simulink model "PlantModelSim"  (R2020a)
settings: Solver=VariableStepAuto  StartTime=0.0  StopTime=30  RelTol=1e-3
values from neighbouring files (symbols this model uses):
  A = [0  0  0  1  0  0  0  0  0  0  0  0 ... (first row only)    [LQR.m]    (also in LQR_Goal_1.m; Naman_LQR_Working.m; PlantModel.m = [0  0  0  1  0  0  0  0  0  0  0  0;      0  0  0  0  1  0  )
  B = [0      0       0       0 ... (first row only)    [LQR.m]    (also in LQR_Goal_1.m; Naman_LQR_Working.m; PlantModel.m = [0 0 0 0;      0 0 0 0;      0 0 0 0;      0 0 0 0;      0 0)
  C = [1 0 0 0 0 0 0 0 0 0 0 0 ... (first row only)    [LQR.m]    (also in LQR_Goal_1.m; Naman_LQR_Working.m; PlantModel.m = [1 0 0 0 0 0 0 0 0 0 0 0;      0 1 0 0 0 0 0 0 0 0 0 0;     )
  D = zeros(6,4)    [LQR.m]    (also in LQR_Goal_1.m; Naman_LQR_Working.m; PlantModel.m)
  g = 9.81    [LQR.m]    (also in LQR_Goal_1.m; Naman_LQR_Working.m; PlantModel.m)
  initialCondition = [x0, y0, z0, xdot0, ydot0, zdot0, phi0, theta0, psi0, phidot0, thetadot0, psidot0]    [PlantModel.m]
  Ix = 4.856*10^-3    (= 0.004856)    [LQR.m]    (also in LQR_Goal_1.m; Naman_LQR_Working.m; PlantModel.m)
  Iy = 4.856*10^-3    (= 0.004856)    [LQR.m]    (also in LQR_Goal_1.m; Naman_LQR_Working.m; PlantModel.m)
  Iz = 8.801*10^-3    (= 0.008801)    [LQR.m]    (also in LQR_Goal_1.m; Naman_LQR_Working.m; PlantModel.m)
  kdp = 0.1    [PlantModel.m]
  kdps = 0.0486    [PlantModel.m]
  kdt = 0.1    [PlantModel.m]
  kdz = 2.9031    [PlantModel.m]
  kpp = 0.4754    [PlantModel.m]
  kpps = 0.0901    [PlantModel.m]
  kpt = 0.4754    [PlantModel.m]
  kpz = 4.0670    (= 4.067)    [PlantModel.m]
  m = 0.468    [LQR.m]    (also in LQR_Goal_1.m; Naman_LQR_Working.m; PlantModel.m)
  phi0 = X0(7)    [LQR_Goal_1.m]    (also in PlantModel.m = 0)
  phidot0 = X0(10)    [LQR_Goal_1.m]    (also in PlantModel.m = 0)
  psi0 = X0(9)    [LQR_Goal_1.m]    (also in PlantModel.m = 0)
  psidot0 = X0(12)    [LQR_Goal_1.m]    (also in PlantModel.m = 0)
  sysd = c2d(sys, 1/100)    [PlantModel.m]
  theta0 = X0(8)    [LQR_Goal_1.m]    (also in PlantModel.m = 0)
  thetadot0 = X0(11)    [LQR_Goal_1.m]    (also in PlantModel.m = 0)
  x0 = X0(1)    [LQR_Goal_1.m]    (also in PlantModel.m = 0)
  x_d = 0    [LQR.m]    (also in PlantModel.m = 1)
  xdot0 = X0(4)    [LQR_Goal_1.m]    (also in PlantModel.m = 0)
  y0 = X0(2)    [LQR_Goal_1.m]    (also in PlantModel.m = 0)
  y_d = 0    [LQR.m]    (also in PlantModel.m = 1)
  ydot0 = X0(5)    [LQR_Goal_1.m]    (also in PlantModel.m = 0)
  z0 = X0(3)    [LQR_Goal_1.m]    (also in PlantModel.m = 0)
  z_d = 0    [LQR.m]    (also in PlantModel.m = 1)
  zdot0 = X0(6)    [LQR_Goal_1.m]    (also in PlantModel.m = 0)
libraries: simulink x11
settings Model: Creator=Lakshu  LastModifiedBy=Sravan

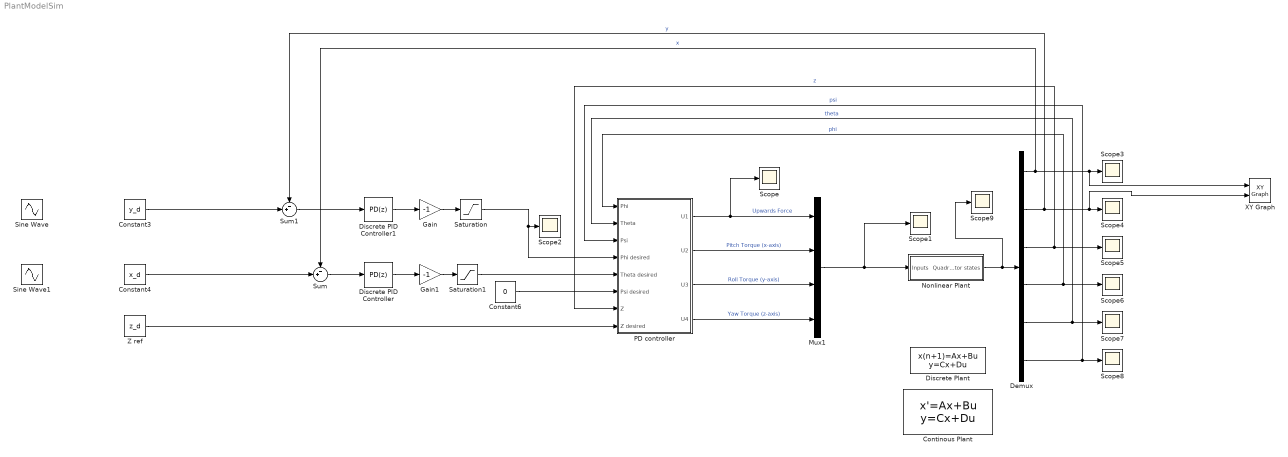
== system PlantModelSim ==
  Constant3 : Constant  Value=y_d
  Constant4 : Constant  Value=x_d
  Constant6 : Constant  Value=0
  Continous Plant : StateSpace  A=A  B=B  C=C  D=D  InitialCondition=initialCondition
  Demux : Demux  Outputs=6
  Discrete PID Controller : simulink/Continuous/PID Controller  Controller=PD  Form=Parallel  TimeDomain=Discrete-time  UseExternalTs=off  SampleTime=-1  IntegratorMethod=Forward Euler  FilterMethod=Forward Euler  ControllerParametersSource=internal  P=-0.0231859221153857  I=-0.00134790003505014  D=-0.0997082443730221  UseFilter=off  N=100  TunerSelectOption=Transfer Function Based (PID Tuner App)  InitialConditionSource=internal  InitialConditionForIntegrator=0  InitialConditionForFilter=0  DifferentiatorICPrevScaledInput=0  ExternalReset=none  TrackingMode=off  Kt=1  LimitOutput=off  UpperSaturationLimit=inf  LowerSaturationLimit=-inf  LinearizeAsGain=off  AntiWindupMode=none  Kb=1  POutMin=[]  POutMax=[]  IOutMin=[]  IOutMax=[]  DOutMin=[]  DOutMax=[]  NOutMin=[]  NOutMax=[]  SumOutMin=[]  SumOutMax=[]  SaturationOutMin=[]  SaturationOutMax=[]  PParamMin=[]  PParamMax=[]  IParamMin=[]  IParamMax=[]  DParamMin=[]  DParamMax=[]  NParamMin=[]  NParamMax=[]  KbParamMin=[]  KbParamMax=[]  KtParamMin=[]  KtParamMax=[]  KbOutMin=[]  KbOutMax=[]  KtOutMin=[]  KtOutMax=[]  IntegratorOutMin=[]  IntegratorOutMax=[]  FilterOutMin=[]  FilterOutMax=[]  SumI1OutMin=[]  SumI1OutMax=[]  SumI2OutMin=[]  SumI2OutMax=[]  SumI3OutMin=[]  SumI3OutMax=[]  SumI4OutMin=[]  SumI4OutMax=[]  SumDOutMin=[]  SumDOutMax=[]  DifferentiatorOutMin=[]  DifferentiatorOutMax=[]  FilterDiffOutCoefMin=[]  FilterDiffOutCoefMax=[]  ReciprocalOutMin=[]  ReciprocalOutMax=[]  SumDenOutMin=[]  SumDenOutMax=[]  SumNumOutMin=[]  SumNumOutMax=[]  DivideOutMin=[]  DivideOutMax=[]  UdiffTsProdOutMin=[]  UdiffTsProdOutMax=[]  NTsProdOutMin=[]  NTsProdOutMax=[]  UintegralTsProdOutMin=[]  UintegralTsProdOutMax=[]  UngainTsProdOutMin=[]  UngainTsProdOutMax=[]  IntegratorContinuousStateAttributes=''  IntegratorStateMustResolveToSignalObject=off  IntegratorRTWStateStorageClass=Auto  FilterContinuousStateAttributes=''  FilterStateMustResolveToSignalObject=off  FilterRTWStateStorageClass=Auto  ParallelPVariant=InternalParameters  IdealPVariant=Disabled  IVariant=Disabled  DVariant=InternalParameters  IntegratorVariant=Disabled  SatVariant=Disabled  AWVariant=Disabled  PCopyVariant=Disabled  TRVariant=Disabled  FdbkBlocksVariant=Forward  IdealPFdbkVariant=Disabled  SatFdbkVariant=Disabled  DerivativeFilterVariant=Differentiator  NVariant=Passthrough  NCopyVariant=Disabled_SignalSpec  FilterICVariant=InternalICsDifferentiator  IntegratorICVariant=Disabled  ExternalResetVariant=Disabled  TRSumVariant=Passthrough  SumFdbkVariant=Disabled  SumVariant=Sum_PD  TsampFilterVariant=InternalTs  TsampNgainVariant=Passthrough  TsampIntegralVariant=Disabled_SignalSpec
  Discrete PID Controller1 : simulink/Continuous/PID Controller  Controller=PD  Form=Parallel  TimeDomain=Discrete-time  UseExternalTs=off  SampleTime=-1  IntegratorMethod=Forward Euler  FilterMethod=Forward Euler  ControllerParametersSource=internal  P=0.0231859221153852  I=0.00134790003505011  D=0.0997082443730201  UseFilter=off  N=100  TunerSelectOption=Transfer Function Based (PID Tuner App)  InitialConditionSource=internal  InitialConditionForIntegrator=0  InitialConditionForFilter=0  DifferentiatorICPrevScaledInput=0  ExternalReset=none  TrackingMode=off  Kt=1  LimitOutput=off  UpperSaturationLimit=inf  LowerSaturationLimit=-inf  LinearizeAsGain=off  AntiWindupMode=none  Kb=1  POutMin=[]  POutMax=[]  IOutMin=[]  IOutMax=[]  DOutMin=[]  DOutMax=[]  NOutMin=[]  NOutMax=[]  SumOutMin=[]  SumOutMax=[]  SaturationOutMin=[]  SaturationOutMax=[]  PParamMin=[]  PParamMax=[]  IParamMin=[]  IParamMax=[]  DParamMin=[]  DParamMax=[]  NParamMin=[]  NParamMax=[]  KbParamMin=[]  KbParamMax=[]  KtParamMin=[]  KtParamMax=[]  KbOutMin=[]  KbOutMax=[]  KtOutMin=[]  KtOutMax=[]  IntegratorOutMin=[]  IntegratorOutMax=[]  FilterOutMin=[]  FilterOutMax=[]  SumI1OutMin=[]  SumI1OutMax=[]  SumI2OutMin=[]  SumI2OutMax=[]  SumI3OutMin=[]  SumI3OutMax=[]  SumI4OutMin=[]  SumI4OutMax=[]  SumDOutMin=[]  SumDOutMax=[]  DifferentiatorOutMin=[]  DifferentiatorOutMax=[]  FilterDiffOutCoefMin=[]  FilterDiffOutCoefMax=[]  ReciprocalOutMin=[]  ReciprocalOutMax=[]  SumDenOutMin=[]  SumDenOutMax=[]  SumNumOutMin=[]  SumNumOutMax=[]  DivideOutMin=[]  DivideOutMax=[]  UdiffTsProdOutMin=[]  UdiffTsProdOutMax=[]  NTsProdOutMin=[]  NTsProdOutMax=[]  UintegralTsProdOutMin=[]  UintegralTsProdOutMax=[]  UngainTsProdOutMin=[]  UngainTsProdOutMax=[]  IntegratorContinuousStateAttributes=''  IntegratorStateMustResolveToSignalObject=off  IntegratorRTWStateStorageClass=Auto  FilterContinuousStateAttributes=''  FilterStateMustResolveToSignalObject=off  FilterRTWStateStorageClass=Auto  ParallelPVariant=InternalParameters  IdealPVariant=Disabled  IVariant=Disabled  DVariant=InternalParameters  IntegratorVariant=Disabled  SatVariant=Disabled  AWVariant=Disabled  PCopyVariant=Disabled  TRVariant=Disabled  FdbkBlocksVariant=Forward  IdealPFdbkVariant=Disabled  SatFdbkVariant=Disabled  DerivativeFilterVariant=Differentiator  NVariant=Passthrough  NCopyVariant=Disabled_SignalSpec  FilterICVariant=InternalICsDifferentiator  IntegratorICVariant=Disabled  ExternalResetVariant=Disabled  TRSumVariant=Passthrough  SumFdbkVariant=Disabled  SumVariant=Sum_PD  TsampFilterVariant=InternalTs  TsampNgainVariant=Passthrough  TsampIntegralVariant=Disabled_SignalSpec
  Discrete Plant : DiscreteStateSpace  A=sysd.A  B=sysd.B  C=sysd.C  D=sysd.D  InitialCondition=initialCondition  SampleTime=.01
  Gain : Gain  Gain=-1
  Gain1 : Gain  Gain=-1
  Mux1 : Mux
  Nonlinear Plant : Subsystem
  PD controller : Subsystem
  Saturation : Saturate  UpperLimit=5*(pi/180)  LowerLimit=-5*(pi/180)
  Saturation1 : Saturate  UpperLimit=5*(pi/180)  LowerLimit=-5*(pi/180)
  Scope{,1..9} (10 alike) : Scope
  Sine Wave : Sin  Amplitude=5  Frequency=.5  SampleTime=0
  Sine Wave1 : Sin  Amplitude=5  Frequency=.5  Phase=pi/2  SampleTime=0
  Sum : Sum  Inputs=-+|
  Sum1 : Sum  Inputs=-+|
  XY Graph : simulink/Sinks/XY Graph  xmin=-7  xmax=7  ymin=-7  ymax=7  st=-1
  Z ref : Constant  Value=z_d
  wires:
  Mux1/1 -> Nonlinear Plant/1(Inputs), Scope1/1
  PD controller/1(U1) -> Scope/1, Mux1/1  "Upwards Force"
  PD controller/2(U2) -> Mux1/2  "Pitch Torque (x-axis)"
  PD controller/3(U3) -> Mux1/3  "Roll Torque (y-axis)"
  PD controller/4(U4) -> Mux1/4  "Yaw Torque (z-axis)"
  Nonlinear Plant/1(Quadrotor states) -> Scope9/1, Demux/1
  Demux/1 -> XY Graph/1, Scope3/1, Sum/1  "x"
  Demux/2 -> XY Graph/2, Scope4/1, Sum1/1  "y"
  Demux/3 -> Scope5/1, PD controller/7(Z)  "z"
  Demux/4 -> Scope6/1, PD controller/1(Phi)  "phi"
  Demux/5 -> Scope7/1, PD controller/2(Theta)  "theta"
  Demux/6 -> Scope8/1, PD controller/3(Psi)  "psi"
  Z ref/1 -> PD controller/8(Z desired)
  Constant6/1 -> PD controller/6(Psi desired)
  Constant4/1 -> Sum/2
  Sum/1 -> Discrete PID Controller/1
  Constant3/1 -> Sum1/2
  Sum1/1 -> Discrete PID Controller1/1
  ? -> ?  "U4"
  Discrete PID Controller1/1 -> Gain/1
  Discrete PID Controller/1 -> Gain1/1
  Saturation/1 -> PD controller/4(Phi desired), Scope2/1
  Saturation1/1 -> PD controller/5(Theta desired)
  Gain/1 -> Saturation/1
  Gain1/1 -> Saturation1/1

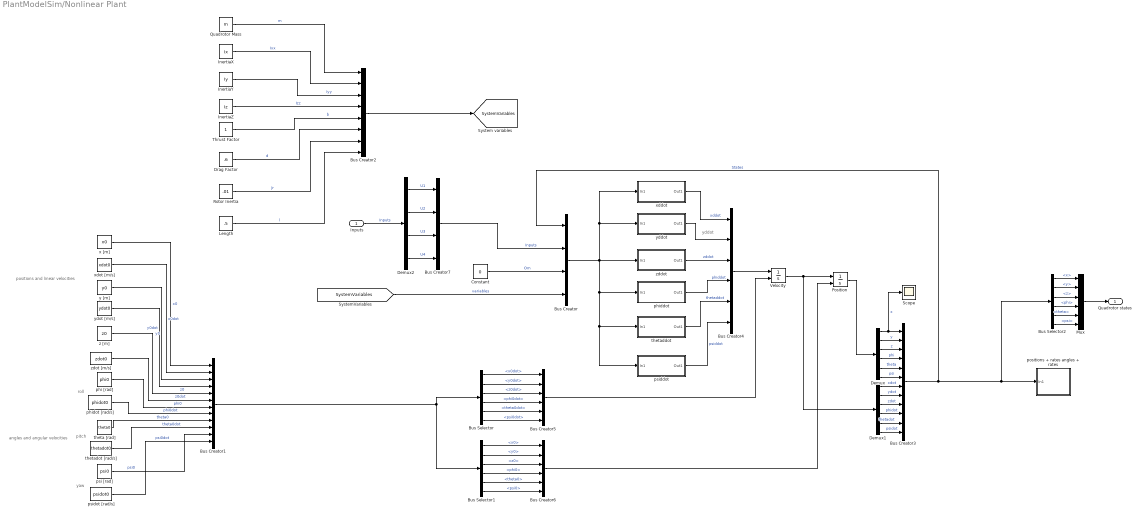
== system PlantModelSim/Nonlinear Plant ==
  note: yddot
  note: positions and linear velocities
  note: pitch
  note: angles and angular velocities
  note: roll
  note: yaw
  Inputs : Inport
  Bus Creator : BusCreator  Inputs=4
  Bus Creator1 : BusCreator  Inputs=12
  Bus Creator2 : BusCreator  Inputs=8
  Bus Creator3 : BusCreator  Inputs=12
  Bus Creator4 : BusCreator  Inputs=6
  Bus Creator5 : BusCreator  Inputs=6
  Bus Creator6 : BusCreator  Inputs=6
  Bus Creator7 : BusCreator  Inputs=4
  Bus Selector : BusSelector  OutputSignals=x0dot,y0dot,z0dot,phi0dot,theta0dot,psi0dot
  Bus Selector1 : BusSelector  OutputSignals=x0,y0,z0,phi0,theta0,psi0
  Bus Selector2 : BusSelector  OutputSignals=x,y,z,phi,theta,psi
  Constant : Constant  Value=0
  Demux : Demux  Outputs=6
  Demux1 : Demux  Outputs=6
  Demux2 : Demux
  Drag Factor : Constant  Value=.6
  InertiaX : Constant  Value=Ix
  InertiaY : Constant  Value=Iy
  InertiaZ : Constant  Value=Iz
  Length : Constant  Value=.5
  Mux : Mux  Inputs=6
  Position : Integrator  InitialConditionSource=external
  Quadrotor Mass : Constant  Value=m
  Rotor Inertia : Constant  Value=.01
  Scope : Scope
  Thrust Factor : Constant
  Velocity : Integrator  InitialConditionSource=external
  phi [rad] : Constant  Value=phi0
  phiddot : Subsystem
  phidot [rad/s] : Constant  Value=phidot0
  positions + rates angles + rates : Subsystem
      mask Display: disp('system states')
  psi [rad] : Constant  Value=psi0
  psiddot : Subsystem
  psidot [rad/s] : Constant  Value=psidot0
  theta [rad] : Constant  Value=theta0
  thetaddot : Subsystem
  thetadot [rad/s] : Constant  Value=thetadot0
  x [m] : Constant  Value=x0
  xddot : Subsystem
  xdot [m/s] : Constant  Value=xdot0
  y [m] : Constant  Value=y0
  yddot : Subsystem
  ydot [m/s] : Constant  Value=ydot0
  z [m] : Constant  Value=z0
  zddot : Subsystem
  zdot [m/s] : Constant  Value=zdot0
  Quadrotor states : Outport
  tag scope: SystemVariables=global
  wires:
  [SystemVariables] -> Bus Creator/4  "variables"
  Bus Creator/1 -> xddot/1(In1), yddot/1(In1), zddot/1(In1), phiddot/1(In1), thetaddot/1(In1), psiddot/1(In1)
  xddot/1(Out1) -> Bus Creator4/1  "xddot"
  yddot/1(Out1) -> Bus Creator4/2
  zddot/1(Out1) -> Bus Creator4/3  "zddot"
  phiddot/1(Out1) -> Bus Creator4/4  "phiddot"
  thetaddot/1(Out1) -> Bus Creator4/5  "thetaddot"
  psiddot/1(Out1) -> Bus Creator4/6  "psiddot"
  Position/1 -> Demux/1
  Bus Creator4/1 -> Velocity/1
  Velocity/1 -> Position/1, Demux1/1
  Bus Creator1/1 -> Bus Selector/1, Bus Selector1/1
  Bus Selector/1 -> Bus Creator5/1  "<x0dot>"
  Bus Selector/2 -> Bus Creator5/2  "<y0dot>"
  Bus Selector/3 -> Bus Creator5/3  "<z0dot>"
  Bus Selector/4 -> Bus Creator5/4  "<phi0dot>"
  Bus Selector/5 -> Bus Creator5/5  "<theta0dot>"
  Bus Selector/6 -> Bus Creator5/6  "<psi0dot>"
  Bus Creator5/1 -> Velocity/2
  Bus Selector1/1 -> Bus Creator6/1  "<x0>"
  Bus Selector1/2 -> Bus Creator6/2  "<y0>"
  Bus Selector1/3 -> Bus Creator6/3  "<z0>"
  Bus Selector1/4 -> Bus Creator6/4  "<phi0>"
  Bus Selector1/5 -> Bus Creator6/5  "<theta0>"
  Bus Selector1/6 -> Bus Creator6/6  "<psi0>"
  Bus Creator6/1 -> Position/2
  Demux/1 -> Scope/1, Bus Creator3/1  "x"
  Demux/2 -> Bus Creator3/2  "y"
  Demux/3 -> Bus Creator3/3  "z"
  Demux/4 -> Bus Creator3/4  "phi"
  Demux/5 -> Bus Creator3/5  "theta"
  Demux/6 -> Bus Creator3/6  "psi"
  Demux1/1 -> Bus Creator3/7  "xdot"
  Demux1/2 -> Bus Creator3/8  "ydot"
  Demux1/3 -> Bus Creator3/9  "zdot"
  Demux1/4 -> Bus Creator3/10  "phidot"
  Demux1/5 -> Bus Creator3/11  "thetadot"
  Demux1/6 -> Bus Creator3/12  "psidot"
  Bus Creator3/1 -> Bus Selector2/1, positions + rates angles + rates/1(In1), Bus Creator/1  "States"
  ydot [m/s]/1 -> Bus Creator1/4  "y0dot"
  psidot [rad/s]/1 -> Bus Creator1/12  "psi0dot"
  x [m]/1 -> Bus Creator1/1  "x0"
  phidot [rad/s]/1 -> Bus Creator1/8  "phi0dot"
  phi [rad]/1 -> Bus Creator1/7  "phi0"
  zdot [m/s]/1 -> Bus Creator1/6  "z0dot"
  y [m]/1 -> Bus Creator1/3  "y0"
  theta [rad]/1 -> Bus Creator1/9  "theta0"
  thetadot [rad/s]/1 -> Bus Creator1/10  "theta0dot"
  z [m]/1 -> Bus Creator1/5  "z0"
  psi [rad]/1 -> Bus Creator1/11  "psi0"
  xdot [m/s]/1 -> Bus Creator1/2  "x0dot"
  Rotor Inertia/1 -> Bus Creator2/7  "Jr"
  Length/1 -> Bus Creator2/8  "l"
  InertiaX/1 -> Bus Creator2/2  "Ixx"
  Drag Factor/1 -> Bus Creator2/6  "d"
  Quadrotor Mass/1 -> Bus Creator2/1  "m"
  Bus Creator2/1 -> [SystemVariables]
  InertiaZ/1 -> Bus Creator2/4  "Izz"
  InertiaY/1 -> Bus Creator2/3  "Iyy"
  Thrust Factor/1 -> Bus Creator2/5  "b"
  Bus Creator7/1 -> Bus Creator/2  "Inputs"
  Constant/1 -> Bus Creator/3  "Om"
  Demux2/1 -> Bus Creator7/1  "U1"
  Demux2/2 -> Bus Creator7/2  "U2"
  Demux2/3 -> Bus Creator7/3  "U3"
  Demux2/4 -> Bus Creator7/4  "U4"
  Inputs/1 -> Demux2/1  "Inputs"
  Bus Selector2/1 -> Mux/1  "<x>"
  Bus Selector2/2 -> Mux/2  "<y>"
  Bus Selector2/3 -> Mux/3  "<z>"
  Bus Selector2/4 -> Mux/4  "<phi>"
  Bus Selector2/5 -> Mux/5  "<theta>"
  Bus Selector2/6 -> Mux/6  "<psi>"
  Mux/1 -> Quadrotor states/1

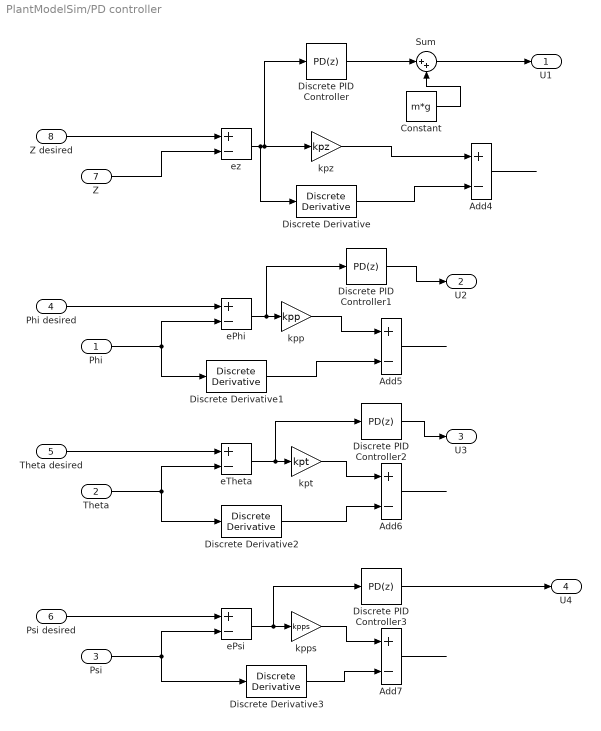
== system PlantModelSim/PD controller ==
  Phi : Inport
  Theta : Inport  Port=2
  Psi : Inport  Port=3
  Phi desired : Inport  Port=4
  Theta desired : Inport  Port=5
  Psi desired : Inport  Port=6
  Z : Inport  Port=7
  Z desired : Inport  Port=8
  Add{4..7} (4 alike) : Sum  Inputs=+-
  Constant : Constant  Value=m*g
  Discrete Derivative : simulink/Discrete/Discrete Derivative  gainval=kdz  ICPrevScaledInput=0.0  OutMin=[]  OutMax=[]  OutDataType=fixdt(1, 16)  OutScaling=2^-10  DoSatur=off
  Discrete Derivative1 : simulink/Discrete/Discrete Derivative  gainval=kdp  ICPrevScaledInput=0.0  OutMin=[]  OutMax=[]  OutDataType=fixdt(1, 16)  OutScaling=2^-10  DoSatur=off
  Discrete Derivative2 : simulink/Discrete/Discrete Derivative  gainval=kdt  ICPrevScaledInput=0.0  OutMin=[]  OutMax=[]  OutDataType=fixdt(1, 16)  OutScaling=2^-10  DoSatur=off
  Discrete Derivative3 : simulink/Discrete/Discrete Derivative  gainval=kdz  ICPrevScaledInput=kdps  OutMin=[]  OutMax=[]  OutDataType=fixdt(1, 16)  OutScaling=2^-10  DoSatur=off
  Discrete PID Controller : simulink/Continuous/PID Controller  Controller=PD  Form=Parallel  TimeDomain=Discrete-time  UseExternalTs=off  SampleTime=-1  IntegratorMethod=Forward Euler  FilterMethod=Forward Euler  ControllerParametersSource=internal  P=kpz  I=1  D=kdz  UseFilter=off  N=10  TunerSelectOption=Transfer Function Based (PID Tuner App)  InitialConditionSource=internal  InitialConditionForIntegrator=0  InitialConditionForFilter=0  DifferentiatorICPrevScaledInput=0  ExternalReset=none  TrackingMode=off  Kt=1  LimitOutput=off  UpperSaturationLimit=inf  LowerSaturationLimit=-inf  LinearizeAsGain=off  AntiWindupMode=none  Kb=1  POutMin=[]  POutMax=[]  IOutMin=[]  IOutMax=[]  DOutMin=[]  DOutMax=[]  NOutMin=[]  NOutMax=[]  SumOutMin=[]  SumOutMax=[]  SaturationOutMin=[]  SaturationOutMax=[]  PParamMin=[]  PParamMax=[]  IParamMin=[]  IParamMax=[]  DParamMin=[]  DParamMax=[]  NParamMin=[]  NParamMax=[]  KbParamMin=[]  KbParamMax=[]  KtParamMin=[]  KtParamMax=[]  KbOutMin=[]  KbOutMax=[]  KtOutMin=[]  KtOutMax=[]  IntegratorOutMin=[]  IntegratorOutMax=[]  FilterOutMin=[]  FilterOutMax=[]  SumI1OutMin=[]  SumI1OutMax=[]  SumI2OutMin=[]  SumI2OutMax=[]  SumI3OutMin=[]  SumI3OutMax=[]  SumI4OutMin=[]  SumI4OutMax=[]  SumDOutMin=[]  SumDOutMax=[]  DifferentiatorOutMin=[]  DifferentiatorOutMax=[]  FilterDiffOutCoefMin=[]  FilterDiffOutCoefMax=[]  ReciprocalOutMin=[]  ReciprocalOutMax=[]  SumDenOutMin=[]  SumDenOutMax=[]  SumNumOutMin=[]  SumNumOutMax=[]  DivideOutMin=[]  DivideOutMax=[]  UdiffTsProdOutMin=[]  UdiffTsProdOutMax=[]  NTsProdOutMin=[]  NTsProdOutMax=[]  UintegralTsProdOutMin=[]  UintegralTsProdOutMax=[]  UngainTsProdOutMin=[]  UngainTsProdOutMax=[]  IntegratorContinuousStateAttributes=''  IntegratorStateMustResolveToSignalObject=off  IntegratorRTWStateStorageClass=Auto  FilterContinuousStateAttributes=''  FilterStateMustResolveToSignalObject=off  FilterRTWStateStorageClass=Auto  ParallelPVariant=InternalParameters  IdealPVariant=Disabled  IVariant=Disabled  DVariant=InternalParameters  IntegratorVariant=Disabled  SatVariant=Disabled  AWVariant=Disabled  PCopyVariant=Disabled  TRVariant=Disabled  FdbkBlocksVariant=Forward  IdealPFdbkVariant=Disabled  SatFdbkVariant=Disabled  DerivativeFilterVariant=Differentiator  NVariant=Passthrough  NCopyVariant=Disabled_SignalSpec  FilterICVariant=InternalICsDifferentiator  IntegratorICVariant=Disabled  ExternalResetVariant=Disabled  TRSumVariant=Passthrough  SumFdbkVariant=Disabled  SumVariant=Sum_PD  TsampFilterVariant=InternalTs  TsampNgainVariant=Passthrough  TsampIntegralVariant=Disabled_SignalSpec
  Discrete PID Controller1 : simulink/Continuous/PID Controller  Controller=PD  Form=Parallel  TimeDomain=Discrete-time  UseExternalTs=off  SampleTime=-1  IntegratorMethod=Forward Euler  FilterMethod=Forward Euler  ControllerParametersSource=internal  P=kpp  I=1  D=kdp  UseFilter=off  N=10  TunerSelectOption=Transfer Function Based (PID Tuner App)  InitialConditionSource=internal  InitialConditionForIntegrator=0  InitialConditionForFilter=0  DifferentiatorICPrevScaledInput=0  ExternalReset=none  TrackingMode=off  Kt=1  LimitOutput=off  UpperSaturationLimit=inf  LowerSaturationLimit=-inf  LinearizeAsGain=off  AntiWindupMode=none  Kb=1  POutMin=[]  POutMax=[]  IOutMin=[]  IOutMax=[]  DOutMin=[]  DOutMax=[]  NOutMin=[]  NOutMax=[]  SumOutMin=[]  SumOutMax=[]  SaturationOutMin=[]  SaturationOutMax=[]  PParamMin=[]  PParamMax=[]  IParamMin=[]  IParamMax=[]  DParamMin=[]  DParamMax=[]  NParamMin=[]  NParamMax=[]  KbParamMin=[]  KbParamMax=[]  KtParamMin=[]  KtParamMax=[]  KbOutMin=[]  KbOutMax=[]  KtOutMin=[]  KtOutMax=[]  IntegratorOutMin=[]  IntegratorOutMax=[]  FilterOutMin=[]  FilterOutMax=[]  SumI1OutMin=[]  SumI1OutMax=[]  SumI2OutMin=[]  SumI2OutMax=[]  SumI3OutMin=[]  SumI3OutMax=[]  SumI4OutMin=[]  SumI4OutMax=[]  SumDOutMin=[]  SumDOutMax=[]  DifferentiatorOutMin=[]  DifferentiatorOutMax=[]  FilterDiffOutCoefMin=[]  FilterDiffOutCoefMax=[]  ReciprocalOutMin=[]  ReciprocalOutMax=[]  SumDenOutMin=[]  SumDenOutMax=[]  SumNumOutMin=[]  SumNumOutMax=[]  DivideOutMin=[]  DivideOutMax=[]  UdiffTsProdOutMin=[]  UdiffTsProdOutMax=[]  NTsProdOutMin=[]  NTsProdOutMax=[]  UintegralTsProdOutMin=[]  UintegralTsProdOutMax=[]  UngainTsProdOutMin=[]  UngainTsProdOutMax=[]  IntegratorContinuousStateAttributes=''  IntegratorStateMustResolveToSignalObject=off  IntegratorRTWStateStorageClass=Auto  FilterContinuousStateAttributes=''  FilterStateMustResolveToSignalObject=off  FilterRTWStateStorageClass=Auto  ParallelPVariant=InternalParameters  IdealPVariant=Disabled  IVariant=Disabled  DVariant=InternalParameters  IntegratorVariant=Disabled  SatVariant=Disabled  AWVariant=Disabled  PCopyVariant=Disabled  TRVariant=Disabled  FdbkBlocksVariant=Forward  IdealPFdbkVariant=Disabled  SatFdbkVariant=Disabled  DerivativeFilterVariant=Differentiator  NVariant=Passthrough  NCopyVariant=Disabled_SignalSpec  FilterICVariant=InternalICsDifferentiator  IntegratorICVariant=Disabled  ExternalResetVariant=Disabled  TRSumVariant=Passthrough  SumFdbkVariant=Disabled  SumVariant=Sum_PD  TsampFilterVariant=InternalTs  TsampNgainVariant=Passthrough  TsampIntegralVariant=Disabled_SignalSpec
  Discrete PID Controller2 : simulink/Continuous/PID Controller  Controller=PD  Form=Parallel  TimeDomain=Discrete-time  UseExternalTs=off  SampleTime=-1  IntegratorMethod=Forward Euler  FilterMethod=Forward Euler  ControllerParametersSource=internal  P=kpt  I=1  D=kdt  UseFilter=off  N=10  TunerSelectOption=Transfer Function Based (PID Tuner App)  InitialConditionSource=internal  InitialConditionForIntegrator=0  InitialConditionForFilter=0  DifferentiatorICPrevScaledInput=0  ExternalReset=none  TrackingMode=off  Kt=1  LimitOutput=off  UpperSaturationLimit=inf  LowerSaturationLimit=-inf  LinearizeAsGain=off  AntiWindupMode=none  Kb=1  POutMin=[]  POutMax=[]  IOutMin=[]  IOutMax=[]  DOutMin=[]  DOutMax=[]  NOutMin=[]  NOutMax=[]  SumOutMin=[]  SumOutMax=[]  SaturationOutMin=[]  SaturationOutMax=[]  PParamMin=[]  PParamMax=[]  IParamMin=[]  IParamMax=[]  DParamMin=[]  DParamMax=[]  NParamMin=[]  NParamMax=[]  KbParamMin=[]  KbParamMax=[]  KtParamMin=[]  KtParamMax=[]  KbOutMin=[]  KbOutMax=[]  KtOutMin=[]  KtOutMax=[]  IntegratorOutMin=[]  IntegratorOutMax=[]  FilterOutMin=[]  FilterOutMax=[]  SumI1OutMin=[]  SumI1OutMax=[]  SumI2OutMin=[]  SumI2OutMax=[]  SumI3OutMin=[]  SumI3OutMax=[]  SumI4OutMin=[]  SumI4OutMax=[]  SumDOutMin=[]  SumDOutMax=[]  DifferentiatorOutMin=[]  DifferentiatorOutMax=[]  FilterDiffOutCoefMin=[]  FilterDiffOutCoefMax=[]  ReciprocalOutMin=[]  ReciprocalOutMax=[]  SumDenOutMin=[]  SumDenOutMax=[]  SumNumOutMin=[]  SumNumOutMax=[]  DivideOutMin=[]  DivideOutMax=[]  UdiffTsProdOutMin=[]  UdiffTsProdOutMax=[]  NTsProdOutMin=[]  NTsProdOutMax=[]  UintegralTsProdOutMin=[]  UintegralTsProdOutMax=[]  UngainTsProdOutMin=[]  UngainTsProdOutMax=[]  IntegratorContinuousStateAttributes=''  IntegratorStateMustResolveToSignalObject=off  IntegratorRTWStateStorageClass=Auto  FilterContinuousStateAttributes=''  FilterStateMustResolveToSignalObject=off  FilterRTWStateStorageClass=Auto  ParallelPVariant=InternalParameters  IdealPVariant=Disabled  IVariant=Disabled  DVariant=InternalParameters  IntegratorVariant=Disabled  SatVariant=Disabled  AWVariant=Disabled  PCopyVariant=Disabled  TRVariant=Disabled  FdbkBlocksVariant=Forward  IdealPFdbkVariant=Disabled  SatFdbkVariant=Disabled  DerivativeFilterVariant=Differentiator  NVariant=Passthrough  NCopyVariant=Disabled_SignalSpec  FilterICVariant=InternalICsDifferentiator  IntegratorICVariant=Disabled  ExternalResetVariant=Disabled  TRSumVariant=Passthrough  SumFdbkVariant=Disabled  SumVariant=Sum_PD  TsampFilterVariant=InternalTs  TsampNgainVariant=Passthrough  TsampIntegralVariant=Disabled_SignalSpec
  Discrete PID Controller3 : simulink/Continuous/PID Controller  Controller=PD  Form=Parallel  TimeDomain=Discrete-time  UseExternalTs=off  SampleTime=-1  IntegratorMethod=Forward Euler  FilterMethod=Forward Euler  ControllerParametersSource=internal  P=kpps  I=1  D=kdps  UseFilter=off  N=10  TunerSelectOption=Transfer Function Based (PID Tuner App)  InitialConditionSource=internal  InitialConditionForIntegrator=0  InitialConditionForFilter=0  DifferentiatorICPrevScaledInput=0  ExternalReset=none  TrackingMode=off  Kt=1  LimitOutput=off  UpperSaturationLimit=inf  LowerSaturationLimit=-inf  LinearizeAsGain=off  AntiWindupMode=none  Kb=1  POutMin=[]  POutMax=[]  IOutMin=[]  IOutMax=[]  DOutMin=[]  DOutMax=[]  NOutMin=[]  NOutMax=[]  SumOutMin=[]  SumOutMax=[]  SaturationOutMin=[]  SaturationOutMax=[]  PParamMin=[]  PParamMax=[]  IParamMin=[]  IParamMax=[]  DParamMin=[]  DParamMax=[]  NParamMin=[]  NParamMax=[]  KbParamMin=[]  KbParamMax=[]  KtParamMin=[]  KtParamMax=[]  KbOutMin=[]  KbOutMax=[]  KtOutMin=[]  KtOutMax=[]  IntegratorOutMin=[]  IntegratorOutMax=[]  FilterOutMin=[]  FilterOutMax=[]  SumI1OutMin=[]  SumI1OutMax=[]  SumI2OutMin=[]  SumI2OutMax=[]  SumI3OutMin=[]  SumI3OutMax=[]  SumI4OutMin=[]  SumI4OutMax=[]  SumDOutMin=[]  SumDOutMax=[]  DifferentiatorOutMin=[]  DifferentiatorOutMax=[]  FilterDiffOutCoefMin=[]  FilterDiffOutCoefMax=[]  ReciprocalOutMin=[]  ReciprocalOutMax=[]  SumDenOutMin=[]  SumDenOutMax=[]  SumNumOutMin=[]  SumNumOutMax=[]  DivideOutMin=[]  DivideOutMax=[]  UdiffTsProdOutMin=[]  UdiffTsProdOutMax=[]  NTsProdOutMin=[]  NTsProdOutMax=[]  UintegralTsProdOutMin=[]  UintegralTsProdOutMax=[]  UngainTsProdOutMin=[]  UngainTsProdOutMax=[]  IntegratorContinuousStateAttributes=''  IntegratorStateMustResolveToSignalObject=off  IntegratorRTWStateStorageClass=Auto  FilterContinuousStateAttributes=''  FilterStateMustResolveToSignalObject=off  FilterRTWStateStorageClass=Auto  ParallelPVariant=InternalParameters  IdealPVariant=Disabled  IVariant=Disabled  DVariant=InternalParameters  IntegratorVariant=Disabled  SatVariant=Disabled  AWVariant=Disabled  PCopyVariant=Disabled  TRVariant=Disabled  FdbkBlocksVariant=Forward  IdealPFdbkVariant=Disabled  SatFdbkVariant=Disabled  DerivativeFilterVariant=Differentiator  NVariant=Passthrough  NCopyVariant=Disabled_SignalSpec  FilterICVariant=InternalICsDifferentiator  IntegratorICVariant=Disabled  ExternalResetVariant=Disabled  TRSumVariant=Passthrough  SumFdbkVariant=Disabled  SumVariant=Sum_PD  TsampFilterVariant=InternalTs  TsampNgainVariant=Passthrough  TsampIntegralVariant=Disabled_SignalSpec
  Sum : Sum  Inputs=|++
  ePhi : Sum  Inputs=+-
  ePsi : Sum  Inputs=+-
  eTheta : Sum  Inputs=+-
  ez : Sum  Inputs=+-
  kpp : Gain  Gain=kpp
  kpps : Gain  Gain=kpps
  kpt : Gain  Gain=kpt
  kpz : Gain  Gain=kpz
  U1 : Outport
  U2 : Outport  Port=2
  U3 : Outport  Port=3
  U4 : Outport  Port=4
  wires:
  Phi/1 -> Discrete Derivative1/1, ePhi/2
  Theta/1 -> Discrete Derivative2/1, eTheta/2
  Psi/1 -> Discrete Derivative3/1, ePsi/2
  Phi desired/1 -> ePhi/1
  Theta desired/1 -> eTheta/1
  Psi desired/1 -> ePsi/1
  ePhi/1 -> Discrete PID Controller1/1, kpp/1
  eTheta/1 -> Discrete PID Controller2/1, kpt/1
  ePsi/1 -> Discrete PID Controller3/1, kpps/1
  Z/1 -> ez/2
  Z desired/1 -> ez/1
  ez/1 -> Discrete Derivative/1, Discrete PID Controller/1, kpz/1
  kpz/1 -> Add4/1
  Discrete Derivative/1 -> Add4/2
  kpp/1 -> Add5/1
  Discrete Derivative1/1 -> Add5/2
  Add5/1 -> ?
  kpt/1 -> Add6/1
  Discrete Derivative2/1 -> Add6/2
  Add6/1 -> ?
  kpps/1 -> Add7/1
  Discrete Derivative3/1 -> Add7/2
  Add7/1 -> ?
  Add4/1 -> ?
  Discrete PID Controller1/1 -> U2/1
  Discrete PID Controller2/1 -> U3/1
  Discrete PID Controller3/1 -> U4/1
  Discrete PID Controller/1 -> Sum/1
  Constant/1 -> Sum/2
  Sum/1 -> U1/1

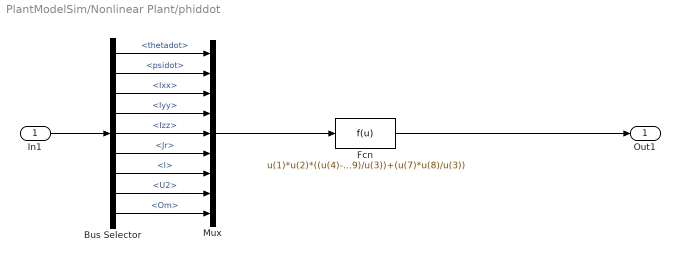
== system PlantModelSim/Nonlinear Plant/phiddot ==
  In1 : Inport
  Bus Selector : BusSelector  OutputSignals=States.thetadot,States.psidot,variables.Ixx,variables.Iyy,variables.Izz,variables.Jr,variables.l,Inputs.U2,Om
  Fcn : Fcn  Expr=u(1)*u(2)*((u(4)-u(5))/u(3))-(u(6)*u(1)*u(9)/u(3))+(u(7)*u(8)/u(3))
  Mux : Mux  Inputs=9
  Out1 : Outport
  wires:
  Bus Selector/7 -> Mux/7  "<l>"
  Mux/1 -> Fcn/1
  Bus Selector/3 -> Mux/3  "<Ixx>"
  Bus Selector/8 -> Mux/8  "<U2>"
  Bus Selector/5 -> Mux/5  "<Izz>"
  Bus Selector/4 -> Mux/4  "<Iyy>"
  Bus Selector/2 -> Mux/2  "<psidot>"
  Bus Selector/1 -> Mux/1  "<thetadot>"
  In1/1 -> Bus Selector/1
  Bus Selector/9 -> Mux/9  "<Om>"
  Fcn/1 -> Out1/1
  Bus Selector/6 -> Mux/6  "<Jr>"

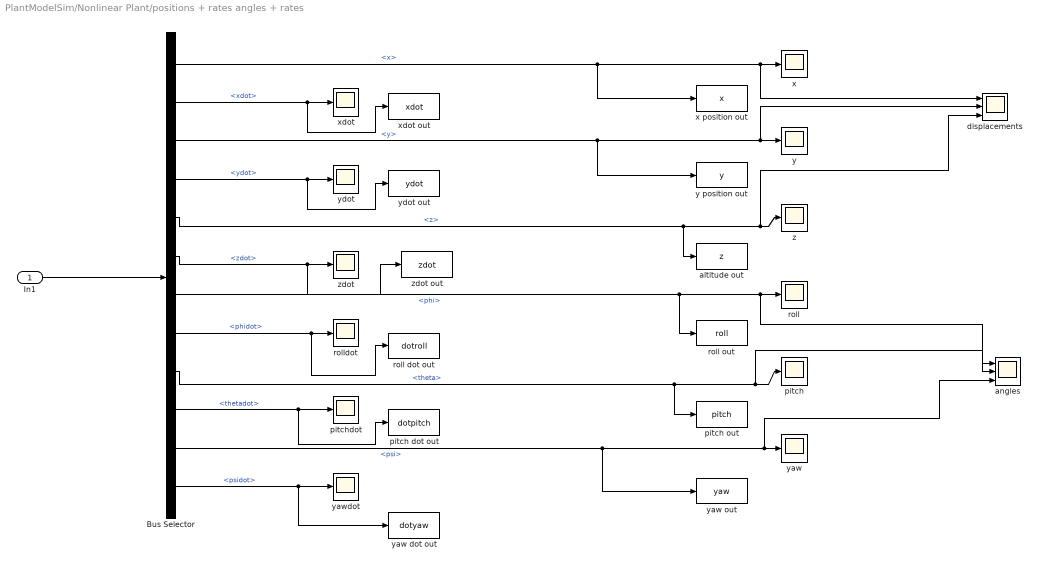
== system PlantModelSim/Nonlinear Plant/positions + rates angles + rates ==
  In1 : Inport
  Bus Selector : BusSelector  OutputSignals=x,xdot,y,ydot,z,zdot,phi,phidot,theta,thetadot,psi,psidot
  altitude out : ToWorkspace  VariableName=z  SampleTime=-1
  angles : Scope  NumInputPorts=3
  displacements : Scope  NumInputPorts=3
  pitch : Scope
  pitch dot out : ToWorkspace  VariableName=dotpitch  SampleTime=-1
  pitch out : ToWorkspace  VariableName=pitch  SampleTime=-1
  pitchdot : Scope
  roll : Scope
  roll dot out : ToWorkspace  VariableName=dotroll  SampleTime=-1
  roll out : ToWorkspace  VariableName=roll  SampleTime=-1
  rolldot : Scope
  x : Scope
  x position out : ToWorkspace  VariableName=x  SampleTime=-1
  xdot : Scope
  xdot out : ToWorkspace  VariableName=xdot  SampleTime=-1
  y : Scope
  y position out : ToWorkspace  VariableName=y  SampleTime=-1
  yaw : Scope
  yaw dot out : ToWorkspace  VariableName=dotyaw  SampleTime=-1
  yaw out : ToWorkspace  VariableName=yaw  SampleTime=-1
  yawdot : Scope
  ydot : Scope
  ydot out : ToWorkspace  VariableName=ydot  SampleTime=-1
  z : Scope
  zdot : Scope
  zdot out : ToWorkspace  VariableName=zdot  SampleTime=-1
  wires:
  Bus Selector/2 -> xdot/1, xdot out/1  "<xdot>"
  Bus Selector/4 -> ydot/1, ydot out/1  "<ydot>"
  Bus Selector/1 -> x position out/1, x/1, displacements/1  "<x>"
  Bus Selector/3 -> y position out/1, y/1, displacements/2  "<y>"
  Bus Selector/12 -> yawdot/1, yaw dot out/1  "<psidot>"
  Bus Selector/11 -> yaw out/1, yaw/1, angles/3  "<psi>"
  In1/1 -> Bus Selector/1
  Bus Selector/10 -> pitchdot/1, pitch dot out/1  "<thetadot>"
  Bus Selector/5 -> altitude out/1, z/1, displacements/3  "<z>"
  Bus Selector/6 -> zdot/1, zdot out/1  "<zdot>"
  Bus Selector/7 -> roll out/1, roll/1, angles/1  "<phi>"
  Bus Selector/8 -> rolldot/1, roll dot out/1  "<phidot>"
  Bus Selector/9 -> pitch out/1, pitch/1, angles/2  "<theta>"

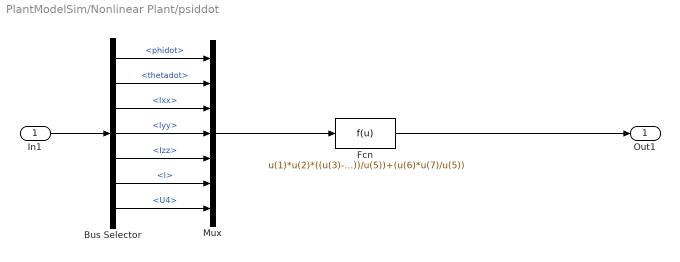
== system PlantModelSim/Nonlinear Plant/psiddot ==
  In1 : Inport
  Bus Selector : BusSelector  OutputSignals=States.phidot,States.thetadot,variables.Ixx,variables.Iyy,variables.Izz,variables.l,Inputs.U4
  Fcn : Fcn  Expr=u(1)*u(2)*((u(3)-u(4))/u(5))+(u(6)*u(7)/u(5))
  Mux : Mux  Inputs=7
  Out1 : Outport
  wires:
  Fcn/1 -> Out1/1
  Mux/1 -> Fcn/1
  In1/1 -> Bus Selector/1
  Bus Selector/1 -> Mux/1  "<phidot>"
  Bus Selector/2 -> Mux/2  "<thetadot>"
  Bus Selector/3 -> Mux/3  "<Ixx>"
  Bus Selector/4 -> Mux/4  "<Iyy>"
  Bus Selector/5 -> Mux/5  "<Izz>"
  Bus Selector/6 -> Mux/6  "<l>"
  Bus Selector/7 -> Mux/7  "<U4>"

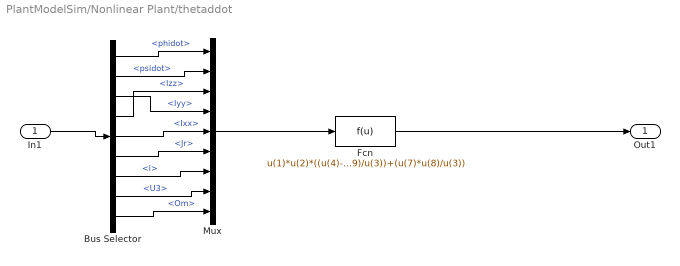
== system PlantModelSim/Nonlinear Plant/thetaddot ==
  In1 : Inport
  Bus Selector : BusSelector  OutputSignals=States.phidot,States.psidot,variables.Iyy,variables.Izz,variables.Ixx,variables.Jr,variables.l,Inputs.U3,Om
  Fcn : Fcn  Expr=u(1)*u(2)*((u(4)-u(5))/u(3))+(u(6)*u(1)*u(9)/u(3))+(u(7)*u(8)/u(3))
  Mux : Mux  Inputs=9
  Out1 : Outport
  wires:
  Bus Selector/1 -> Mux/1  "<phidot>"
  Bus Selector/2 -> Mux/2  "<psidot>"
  Bus Selector/7 -> Mux/7  "<l>"
  Bus Selector/6 -> Mux/6  "<Jr>"
  Bus Selector/3 -> Mux/4  "<Iyy>"
  In1/1 -> Bus Selector/1
  Mux/1 -> Fcn/1
  Fcn/1 -> Out1/1
  Bus Selector/4 -> Mux/3  "<Izz>"
  Bus Selector/5 -> Mux/5  "<Ixx>"
  Bus Selector/8 -> Mux/8  "<U3>"
  Bus Selector/9 -> Mux/9  "<Om>"

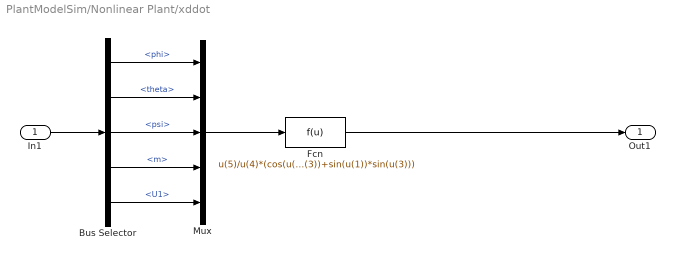
== system PlantModelSim/Nonlinear Plant/xddot ==
  In1 : Inport
  Bus Selector : BusSelector  OutputSignals=States.phi,States.theta,States.psi,variables.m,Inputs.U1
  Fcn : Fcn  Expr=u(5)/u(4)*(cos(u(1))*sin(u(2))*cos(u(3))+sin(u(1))*sin(u(3)))
  Mux : Mux  Inputs=5
  Out1 : Outport
  wires:
  In1/1 -> Bus Selector/1
  Bus Selector/1 -> Mux/1  "<phi>"
  Bus Selector/2 -> Mux/2  "<theta>"
  Bus Selector/3 -> Mux/3  "<psi>"
  Bus Selector/4 -> Mux/4  "<m>"
  Bus Selector/5 -> Mux/5  "<U1>"
  Mux/1 -> Fcn/1
  Fcn/1 -> Out1/1

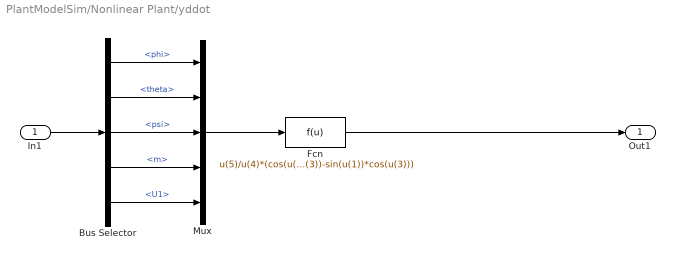
== system PlantModelSim/Nonlinear Plant/yddot ==
  In1 : Inport
  Bus Selector : BusSelector  OutputSignals=States.phi,States.theta,States.psi,variables.m,Inputs.U1
  Fcn : Fcn  Expr=u(5)/u(4)*(cos(u(1))*sin(u(2))*sin(u(3))-sin(u(1))*cos(u(3)))
  Mux : Mux  Inputs=5
  Out1 : Outport
  wires:
  Fcn/1 -> Out1/1
  Mux/1 -> Fcn/1
  Bus Selector/5 -> Mux/5  "<U1>"
  Bus Selector/4 -> Mux/4  "<m>"
  Bus Selector/3 -> Mux/3  "<psi>"
  Bus Selector/2 -> Mux/2  "<theta>"
  Bus Selector/1 -> Mux/1  "<phi>"
  In1/1 -> Bus Selector/1

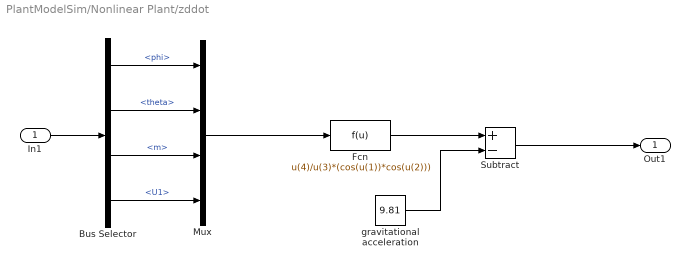
== system PlantModelSim/Nonlinear Plant/zddot ==
  In1 : Inport
  Bus Selector : BusSelector  OutputSignals=States.phi,States.theta,variables.m,Inputs.U1
  Fcn : Fcn  Expr=u(4)/u(3)*(cos(u(1))*cos(u(2)))
  Mux : Mux
  Subtract : Sum  Inputs=+-
  gravitational acceleration : Constant  Value=9.81
  Out1 : Outport
  wires:
  In1/1 -> Bus Selector/1
  Bus Selector/1 -> Mux/1  "<phi>"
  Bus Selector/2 -> Mux/2  "<theta>"
  Mux/1 -> Fcn/1
  Bus Selector/3 -> Mux/3  "<m>"
  Bus Selector/4 -> Mux/4  "<U1>"
  Fcn/1 -> Subtract/1
  gravitational acceleration/1 -> Subtract/2
  Subtract/1 -> Out1/1
